simulink model "Auf7_3"  (R2019a)
settings: Solver=VariableStepAuto  StartTime=0.0  StopTime=60  RelTol=1e-3
undefined symbols (not defined in the file or in its folder): des, gcbh
settings Model: Creator=Naveen  LastModifiedBy=Naveen

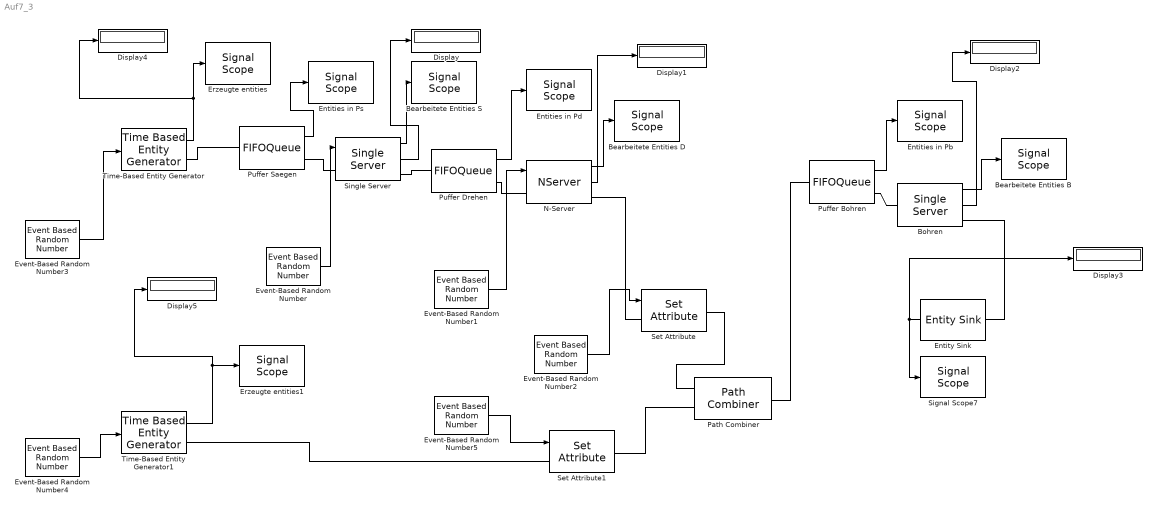
== system Auf7_3 ==
  Bearbeitete Entities B : SignalScope  LoadFcn=des.scope.CallbackSupport('seLoadFcn',gcbh)  StartFcn=des.scope.CallbackSupport('seStartFcn',gcbh)  StopFcn=des.scope.CallbackSupport('seStopFcn',gcbh)
      settings: CopyFcn=des.scope.CallbackSupport('seCopyFcn',gcbh)  DeleteFcn=des.scope.CallbackSupport('seDeleteFcn',gcbh)  PreSaveFcn=des.scope.CallbackSupport('sePreSaveFcn',gcbh)  NameChangeFcn=des.scope.CallbackSupport('seNameChangeFcn',gcbh)  OpenFcn=des.scope.CallbackSupport('seOpenFcn',gcbh)
  Bearbeitete Entities D : SignalScope  LoadFcn=des.scope.CallbackSupport('seLoadFcn',gcbh)  StartFcn=des.scope.CallbackSupport('seStartFcn',gcbh)  StopFcn=des.scope.CallbackSupport('seStopFcn',gcbh)
      settings: CopyFcn=des.scope.CallbackSupport('seCopyFcn',gcbh)  DeleteFcn=des.scope.CallbackSupport('seDeleteFcn',gcbh)  PreSaveFcn=des.scope.CallbackSupport('sePreSaveFcn',gcbh)  NameChangeFcn=des.scope.CallbackSupport('seNameChangeFcn',gcbh)  OpenFcn=des.scope.CallbackSupport('seOpenFcn',gcbh)
  Bearbeitete Entities S : SignalScope  LoadFcn=des.scope.CallbackSupport('seLoadFcn',gcbh)  StartFcn=des.scope.CallbackSupport('seStartFcn',gcbh)  StopFcn=des.scope.CallbackSupport('seStopFcn',gcbh)
      settings: CopyFcn=des.scope.CallbackSupport('seCopyFcn',gcbh)  DeleteFcn=des.scope.CallbackSupport('seDeleteFcn',gcbh)  PreSaveFcn=des.scope.CallbackSupport('sePreSaveFcn',gcbh)  NameChangeFcn=des.scope.CallbackSupport('seNameChangeFcn',gcbh)  OpenFcn=des.scope.CallbackSupport('seOpenFcn',gcbh)
  Bohren : SingleServer  ServiceTimeFrom=Attribute  ServiceTime=ts_sage  StatNumberDeparted=on  StatUtilization=on
      settings: OutputPortMap=o0,o5
  Display{,1..5} (6 alike) : Display
  Entities in Pb : SignalScope  LoadFcn=des.scope.CallbackSupport('seLoadFcn',gcbh)  StartFcn=des.scope.CallbackSupport('seStartFcn',gcbh)  StopFcn=des.scope.CallbackSupport('seStopFcn',gcbh)
      settings: CopyFcn=des.scope.CallbackSupport('seCopyFcn',gcbh)  DeleteFcn=des.scope.CallbackSupport('seDeleteFcn',gcbh)  PreSaveFcn=des.scope.CallbackSupport('sePreSaveFcn',gcbh)  NameChangeFcn=des.scope.CallbackSupport('seNameChangeFcn',gcbh)  OpenFcn=des.scope.CallbackSupport('seOpenFcn',gcbh)
  Entities in Pd : SignalScope  LoadFcn=des.scope.CallbackSupport('seLoadFcn',gcbh)  StartFcn=des.scope.CallbackSupport('seStartFcn',gcbh)  StopFcn=des.scope.CallbackSupport('seStopFcn',gcbh)
      settings: CopyFcn=des.scope.CallbackSupport('seCopyFcn',gcbh)  DeleteFcn=des.scope.CallbackSupport('seDeleteFcn',gcbh)  PreSaveFcn=des.scope.CallbackSupport('sePreSaveFcn',gcbh)  NameChangeFcn=des.scope.CallbackSupport('seNameChangeFcn',gcbh)  OpenFcn=des.scope.CallbackSupport('seOpenFcn',gcbh)
  Entities in Ps : SignalScope  LoadFcn=des.scope.CallbackSupport('seLoadFcn',gcbh)  StartFcn=des.scope.CallbackSupport('seStartFcn',gcbh)  StopFcn=des.scope.CallbackSupport('seStopFcn',gcbh)
      settings: CopyFcn=des.scope.CallbackSupport('seCopyFcn',gcbh)  DeleteFcn=des.scope.CallbackSupport('seDeleteFcn',gcbh)  PreSaveFcn=des.scope.CallbackSupport('sePreSaveFcn',gcbh)  NameChangeFcn=des.scope.CallbackSupport('seNameChangeFcn',gcbh)  OpenFcn=des.scope.CallbackSupport('seOpenFcn',gcbh)
  Entity Sink : EntitySink  StatNumberArrived=on
  Erzeugte entities : SignalScope  LoadFcn=des.scope.CallbackSupport('seLoadFcn',gcbh)  StartFcn=des.scope.CallbackSupport('seStartFcn',gcbh)  StopFcn=des.scope.CallbackSupport('seStopFcn',gcbh)
      settings: CopyFcn=des.scope.CallbackSupport('seCopyFcn',gcbh)  DeleteFcn=des.scope.CallbackSupport('seDeleteFcn',gcbh)  PreSaveFcn=des.scope.CallbackSupport('sePreSaveFcn',gcbh)  NameChangeFcn=des.scope.CallbackSupport('seNameChangeFcn',gcbh)  OpenFcn=des.scope.CallbackSupport('seOpenFcn',gcbh)
  Erzeugte entities1 : SignalScope  LoadFcn=des.scope.CallbackSupport('seLoadFcn',gcbh)  StartFcn=des.scope.CallbackSupport('seStartFcn',gcbh)  StopFcn=des.scope.CallbackSupport('seStopFcn',gcbh)
      settings: CopyFcn=des.scope.CallbackSupport('seCopyFcn',gcbh)  DeleteFcn=des.scope.CallbackSupport('seDeleteFcn',gcbh)  PreSaveFcn=des.scope.CallbackSupport('sePreSaveFcn',gcbh)  NameChangeFcn=des.scope.CallbackSupport('seNameChangeFcn',gcbh)  OpenFcn=des.scope.CallbackSupport('seOpenFcn',gcbh)
  Event-Based Random Number : EventBasedRandomNumber  Distribution=Uniform  minUnif=0.3  maxUnif=1.7
  Event-Based Random Number1 : EventBasedRandomNumber  Distribution=Triangular  minTri=0.5
  Event-Based Random Number2 : EventBasedRandomNumber  Distribution=Uniform  minUnif=0.3  maxUnif=0.7
  Event-Based Random Number3 : EventBasedRandomNumber  minUnif=0.3  maxUnif=1.7
  Event-Based Random Number4 : EventBasedRandomNumber  minUnif=0.4  maxUnif=0.6
  Event-Based Random Number5 : EventBasedRandomNumber  Distribution=Uniform  minUnif=0.4  maxUnif=0.6
  N-Server : NServer  NumberOfServers=2  ServiceTimeFrom=Signal port t  StatNumberDeparted=on  StatUtilization=on
      settings: OutputPortMap=o0,o5
  Path Combiner : PathCombiner  NumberInputPorts=2
  Puffer Bohren : FIFOQueue  Capacity=inf  StatNumberInBlock=on
      settings: OutputPortMap=o1
  Puffer Drehen : FIFOQueue  Capacity=20  StatNumberInBlock=on
      settings: OutputPortMap=o1
  Puffer Saegen : FIFOQueue  Capacity=inf  StatNumberInBlock=on
      settings: OutputPortMap=o1
  Set Attribute : SetAttribute  AttributeName=ServiceTime  AttributeFrom=Signal port  EvaluatedAttributeValue={ []}
  Set Attribute1 : SetAttribute  AttributeName=ServiceTime  AttributeFrom=Signal port  EvaluatedAttributeValue={ []}
  Signal Scope7 : SignalScope  LoadFcn=des.scope.CallbackSupport('seLoadFcn',gcbh)  StartFcn=des.scope.CallbackSupport('seStartFcn',gcbh)  StopFcn=des.scope.CallbackSupport('seStopFcn',gcbh)
      settings: CopyFcn=des.scope.CallbackSupport('seCopyFcn',gcbh)  DeleteFcn=des.scope.CallbackSupport('seDeleteFcn',gcbh)  PreSaveFcn=des.scope.CallbackSupport('sePreSaveFcn',gcbh)  NameChangeFcn=des.scope.CallbackSupport('seNameChangeFcn',gcbh)  OpenFcn=des.scope.CallbackSupport('seOpenFcn',gcbh)
  Single Server : SingleServer  ServiceTimeFrom=Signal port t  ServiceTime=ts_sage  StatNumberDeparted=on  StatUtilization=on
      settings: OutputPortMap=o0,o5
  Time-Based Entity Generator : TimeBasedEntityGenerator  GenerateEntitiesUpon=Intergeneration time from port t  StatNumberDeparted=on
  Time-Based Entity Generator1 : TimeBasedEntityGenerator  GenerateEntitiesUpon=Intergeneration time from port t  StatNumberDeparted=on
  wires:
  Puffer Saegen/1 -> Entities in Ps/1
  Single Server/1 -> Bearbeitete Entities S/1
  Puffer Bohren/1 -> Entities in Pb/1
  Bohren/1 -> Bearbeitete Entities B/1
  Single Server/2 -> Display/1
  Bohren/2 -> Display2/1
  Entity Sink/1 -> Signal Scope7/1, Display3/1
  Time-Based Entity Generator/1 -> Display4/1, Erzeugte entities/1
  Event-Based Random Number1/1 -> N-Server/1
  Puffer Drehen/1 -> Entities in Pd/1
  Event-Based Random Number3/1 -> Time-Based Entity Generator/1
  Event-Based Random Number/1 -> Single Server/1
  N-Server/2 -> Display1/1
  N-Server/1 -> Bearbeitete Entities D/1
  Event-Based Random Number2/1 -> Set Attribute/1
  Event-Based Random Number4/1 -> Time-Based Entity Generator1/1
  Event-Based Random Number5/1 -> Set Attribute1/1
  Time-Based Entity Generator1/1 -> Display5/1, Erzeugte entities1/1
  connections:
  Bohren/RConn1 -- Entity Sink/LConn1
  Single Server/LConn1 -- Puffer Saegen/RConn1
  Puffer Saegen/LConn1 -- Time-Based Entity Generator/RConn1
  Puffer Drehen/LConn1 -- Single Server/RConn1
  N-Server/LConn1 -- Puffer Drehen/RConn1
  Set Attribute1/LConn1 -- Time-Based Entity Generator1/RConn1
  Set Attribute1/RConn1 -- Path Combiner/LConn2
  Path Combiner/RConn1 -- Puffer Bohren/LConn1
  Bohren/LConn1 -- Puffer Bohren/RConn1
  Set Attribute/RConn1 -- Path Combiner/LConn1
  Set Attribute/LConn1 -- N-Server/RConn1
